simulink model "Pump"  (R2021b)
settings: Solver=VariableStepAuto  StartTime=0.0  StopTime=10.0  RelTol=1e-3
undefined symbols (not defined in the file): PumpState
settings Model: Creator=david  LastModifiedBy=david

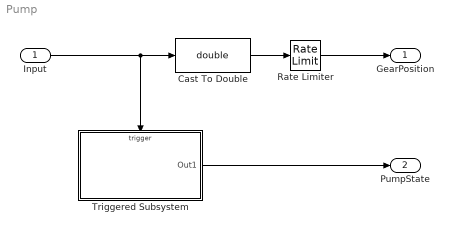
== system Pump ==
  Input : Inport  OutDataTypeStr=Enum: GearPosition
  Cast To Double : DataTypeConversion  OutDataTypeStr=double
  Rate Limiter : RateLimiter  RisingSlewLimit=1/5  FallingSlewLimit=-1/5
  Triggered Subsystem : Subsystem  TreatAsAtomicUnit=on
  GearPosition : Outport
  PumpState : Outport  Port=2  OutDataTypeStr=Enum: PumpState
  wires:
  Input/1 -> Cast To Double/1, Triggered Subsystem/Trigger
  Rate Limiter/1 -> GearPosition/1
  Triggered Subsystem/1(Out1) -> PumpState/1
  Cast To Double/1 -> Rate Limiter/1

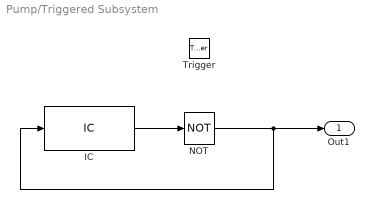
== system Pump/Triggered Subsystem ==
  Trigger : TriggerPort  TriggerType=either  VariantControl=(inherit)
  IC : InitialCondition  Value=PumpState.off
  NOT : Logic  Operator=NOT  AllPortsSameDT=off  OutDataTypeStr=boolean
  Out1 : Outport
  wires:
  NOT/1 -> IC/1, Out1/1
  IC/1 -> NOT/1
